simulink library "etherlab_lib"  (Simulink 7.4)
(part 3 of 4)

      |     sprintf('%s\nM:%i Idx:%s',...
      |             model,master,mat2str(index)))
      settings: AttributesFormatString=|
      | EP8309-1022
      | M:0 Idx:1
      mask Help: web(etherlab_help_path('ep8309.html'), '-helpbrowser');
      mask StyleString: edit,edit,popup(EP8309-1022),edit,edit,edit,checkbox,checkbox,checkbox,checkbox,edit,edit,edit,popup(0..20 mA|4..20 mA),popup(0..20 mA|4..20 mA),popup(Off|50Hz FIR|60Hz FIR|IIR 1|IIR 2|IIR 3|IIR 4|IIR 5|IIR 6|IIR 7|IIR 8),edit,popup(None|Single shaft|Dual shaft),edit,edit,popup(RPM|1/10 RPM|1/100 RPM|Hz|1/10 Hz|1/100 Hz|1/1000 Hz),edit,edit,popup(RPM|1/10 RPM|1/100 RPM|Hz|1/10 Hz|1/100 Hz|1/1000 Hz),checkbox,checkbox,edit,edit,popup(RPM|1/10 RPM|1/100 RPM|Hz|1/10 Hz|1/100 Hz|1/1000 Hz),popup(None|Current|PWM),edit,checkbox,checkbox,popup(Set to default|Ramp to default|Retain last value),edit,edit,edit,edit,edit,edit,edit,edit,popup(Set to default|Ramp to default|Retain last value),edit,edit,popup(0..20 mA|4..20 mA)
      mask CallbackString: ||ep8309().updateRevision()|||||||ep8309.updateAnalogIn||||||||ep8309.updateTacho||||||||||||ep8309.updateAnalogOut||||||||||||||||
      mask TabNameString: Main,Main,Main,Main,Main,Main,Digital,Digital,Digital,Analog Input,Analog Input,Analog Input,Analog Input,Analog Input,Analog Input,Analog Input,Analog Input,Tacho,Tacho,Tacho,Tacho,Tacho,Tacho,Tacho,Tacho,Tacho,Tacho,Tacho,Tacho,Analog Output,Analog Output,Analog Output,Analog Output,Analog Output,Analog Output,Analog Output,Analog Output,Analog Output,Analog Output,Analog Output,Analog Output,Analog Output,Analog Output,Analog Output,Analog Output,Analog Output
      mask Display:
      | port_label('input', 1, 'DigOut')
      | port_label('output', 1, 'DigIn')
  Infrastructure : S-Function  LoadFcn=ekxxxx().checkModelName()  FunctionName=ec_slave3  Parameters=Address,rv.SlaveConfig,rv.PortConfig,debug,tsample  SFunctionModules='ecrt_support'  EnableBusSupport=off  mask(EKxxxx){master=0, index=1, model=EK1100, revision=, vector=off, tsample=0, debug=0}
      mask prompts: index "Slave Index"; model "Device Model"; vector "Vector output"; tsample "Sample Time / Domain"
      mask help:
      | EtherCAT Infrastructure Slaves.
      |
      | Including these slaves (even if they don't have I/Os)
      | will create slave configurations, which will cause them to go into the
      | operational state.
      mask init:
      | Address = EtherCATSlave.formatAddress(master,index,tsample);
      | 
      | rv = ekxxxx(model).configure(vector);
      mask Help: web(etherlab_help_path('ekxxxx.html'), '-helpbrowser')
      mask StyleString: edit,edit,popup(EK1100|EK1100-0030|EK1101|EK1110|EK1122|EK1200|EK1501|EK1501-0010|EK1521|EK1521-0010|EK1541|EK1561|EK1814|EK1818|EK1828|EK1828-0010|CX1100-0004),edit,checkbox,edit,edit
      mask CallbackString: ||ekxxxx().updateRevision()||||
      mask Display: fprintf('%s\nM:%i Idx:%s', model, master, mat2str(index))
